simulink model "PositionControlFuzzy"  (R2022b)
settings: Solver=ode3  StartTime=0.0  StopTime=100.0  FixedStep=Ts  RelTol=1e-3
values from neighbouring files (symbols this model uses):
  th_0 = 0    [parte32.m]
  Ts = 100e-3    (= 0.1)    [comparativa.m]    (also in parte32.m)
  x_0 = 0    [parte32.m]
  y_0 = 0    [parte32.m]
undefined symbols (not defined in the file or in its folder): DiscIntNeverNeededParam, sigbuilder_block
libraries: fuzblock x1
settings Model: PacingRate=10  Creator=Edu  LastModifiedBy=rufo
settings SolverCC: AlgebraicLoopSolver=TrustRegion
settings DataIOCC: ReturnWorkspaceOutputs=off
settings DebuggingCC: UnconnectedInputMsg=warning  UnconnectedOutputMsg=warning  UnconnectedLineMsg=warning  SFMachineParentedDataDiag=warning  ArithmeticOperatorsInVariantConditions=warning
settings ModelReferenceCC: EnableRefExpFcnMdlSchedulingChecks=on
settings SFSimCC: CustomCodeUndefinedFunction=UseInterfaceOnly

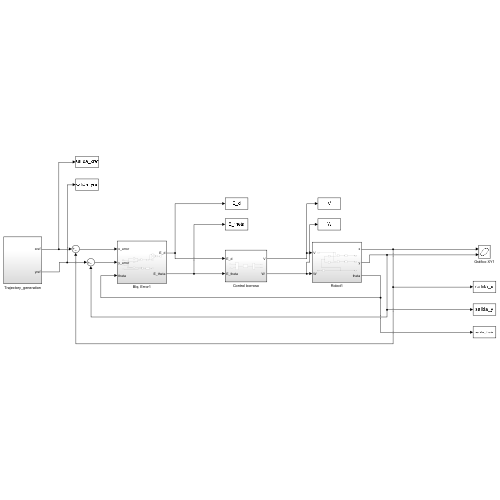
[thumbnail: Simulink's stored preview of the top-level diagram]
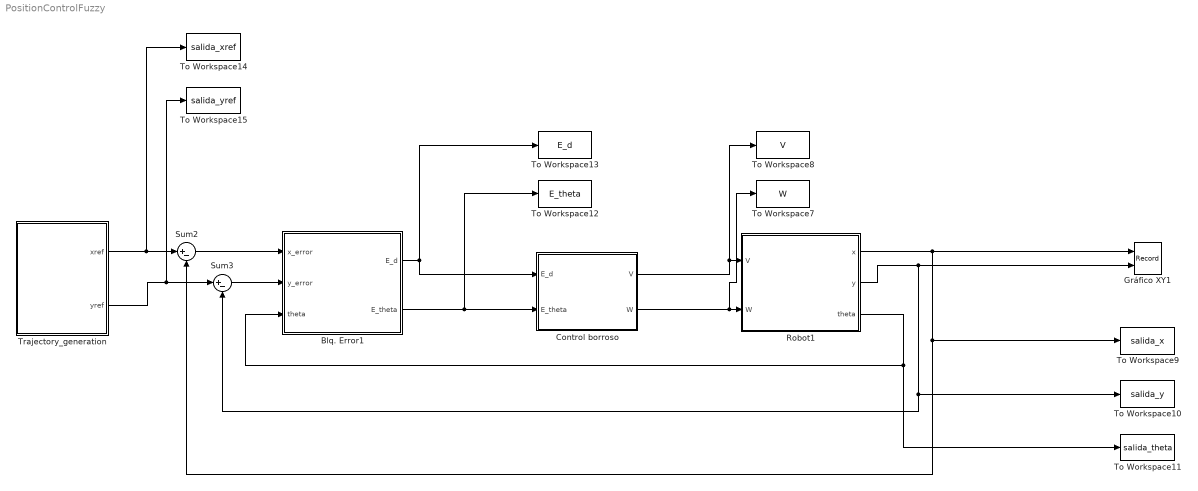
== system PositionControlFuzzy ==
  Blq. Error1 : Subsystem
  Control borroso : Subsystem
  Gráfico XY1 : Record  FileSettingsInternal="{\"entries\":[{\"content\":{\"excelSettings\":{\"content\":{},\"type\":\"Streamout.ExcelSettings\"}},\"type\":\"Streamout.FileSettingStorage\",\"uuid\":\"148716e7-62da-4a17-92fb-a85c316f925a\"}],\"packageUris\":[\"http://schema.mathworks.com/mf0/streamout_blocks/R2020a\"],\"version\":\"1.0\"}"  Layout=[1 1]  SignalsInternal="{\"entries\":[{\"content\":{\"signals\":[{\"content\":{\"blockPath\":[\"PositionControlFuzzy/Gráfico XY1\"],\"channel\":[],\"dimensions\":[1],\"domain\":\"PositionControlFuzzy/Grￃﾡfico XY1\",\"lineColor\":\"#a2142f\",\"plots\":[1],\"port\":1,\"sid\":[\"\"],\"signalID\":1359,\"signalName\":\"Robot1:1\"},\"type\":\"RecordBlkView.Signal\",\"uuid\":\"64a1cd59-4d77-4e73-8dd8-b24fff99f81d\"},{\"content\":{\"blockPath\":[\"PositionControlFuzzy/Gráfico XY1\"],\"channel\":[],\"dimensions\":[1],\"domain\":\"PositionControlFuzzy/Grￃﾡfico XY1\",\"lineColor\":\"#139fff\",\"plots\":[1],\"port\":2,\"sid\":[\"\"],\"signalID\":1363,\"signalName\":\"Robot1:2\"},\"type\":\"RecordBlkView.Signal\",\"uuid\":\"bc7211c2-bf92-4b6c-aa6f-eb73f9fcbfea\"}]},\"type\":\"RecordBlkView.InputSignals\",\"uuid\":\"ff4ee394-39ff-4ff1-a002-becb146826f1\"}],\"packageUris\":[\"http://schema.mathworks.com/mf0/streamout_blocks/R2020a\"],\"version\":\"1.0\"}"  VisualizationBindings="{\"xyplotplugin\":{\"info\":[{\"series\":[{\"bindingParametersList\":[{\"parameter\":\"X-Axis\",\"signalID\":1359,\"signalName\":\"Robot1:1\"},{\"parameter\":\"Y-Axis\",\"signalID\":1363,\"signalName\":\"Robot1:2\"}],\"seriesID\":12570}],\"subplotID\":1}]}}"  CompatibilityTag=XY  st=-1
  Robot1 : Subsystem
  Sum2 : Sum  Inputs=|+-
  Sum3 : Sum  Inputs=|+-
  To Workspace10 : ToWorkspace  VariableName=salida_y  SaveFormat=Structure With Time  SampleTime=-1
  To Workspace11 : ToWorkspace  VariableName=salida_theta  SaveFormat=Structure With Time  SampleTime=-1
  To Workspace12 : ToWorkspace  VariableName=E_theta  SaveFormat=Structure With Time  SampleTime=-1
  To Workspace13 : ToWorkspace  VariableName=E_d  SaveFormat=Structure With Time  SampleTime=-1
  To Workspace14 : ToWorkspace  VariableName=salida_xref  SaveFormat=Structure With Time  SampleTime=-1
  To Workspace15 : ToWorkspace  VariableName=salida_yref  SaveFormat=Structure With Time  SampleTime=-1
  To Workspace7 : ToWorkspace  VariableName=W  SaveFormat=Structure With Time  SampleTime=-1
  To Workspace8 : ToWorkspace  VariableName=V  SaveFormat=Structure With Time  SampleTime=-1
  To Workspace9 : ToWorkspace  VariableName=salida_x  SaveFormat=Structure With Time  SampleTime=-1
  Trajectory_generation : Subsystem
  wires:
  Trajectory_generation/2(yref) -> To Workspace15/1, Sum3/1
  Blq. Error1/1(E_d) -> Control borroso/1("E_d "), To Workspace13/1
  Trajectory_generation/1(xref) -> To Workspace14/1, Sum2/1
  Robot1/2(y) -> Gráfico XY1/2, To Workspace10/1, Sum3/2
  Sum2/1 -> Blq. Error1/1(x_error)
  Blq. Error1/2(E_theta) -> Control borroso/2(E_theta), To Workspace12/1
  Robot1/3(theta) -> Blq. Error1/3(theta), To Workspace11/1
  Robot1/1(x) -> Gráfico XY1/1, To Workspace9/1, Sum2/2
  Sum3/1 -> Blq. Error1/2(y_error)
  Control borroso/1(V) -> To Workspace8/1, Robot1/1(V)
  Control borroso/2("W ") -> To Workspace7/1, Robot1/2(W)

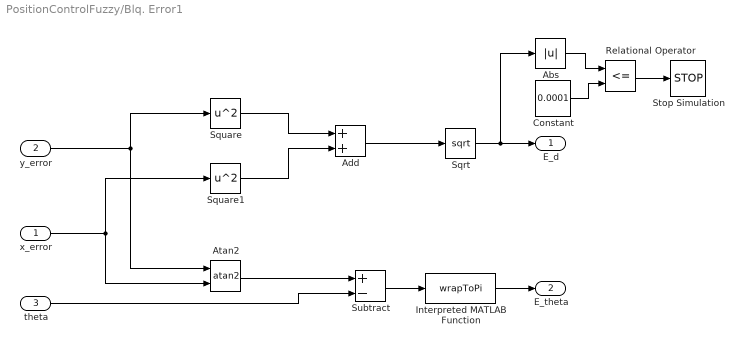
== system PositionControlFuzzy/Blq. Error1 ==
  x_error : Inport
  y_error : Inport  Port=2
  theta : Inport  Port=3
  Abs : Abs  SaturateOnIntegerOverflow=off
  Add : Sum
  Atan2 : Trigonometry  Operator=atan2
  Constant : Constant  Value=0.0001
  Interpreted MATLAB Function : MATLABFcn  MATLABFcn=wrapToPi
  Relational Operator : RelationalOperator  Operator=<=  OutDataTypeStr=boolean  RndMeth=Simplest  InputSameDT=off
  Sqrt : Sqrt
  Square : Math  Operator=square  SignedPower=on
  Square1 : Math  Operator=square  SignedPower=on
  Stop Simulation : Stop
  Subtract : Sum  Inputs=+-  OutMin=[-3.14]  OutMax=[3.14]
  E_d : Outport  VectorParamsAs1DForOutWhenUnconnected=off
  E_theta : Outport  Port=2  OutMin=[-pi]  OutMax=[pi]  VectorParamsAs1DForOutWhenUnconnected=off
  wires:
  y_error/1 -> Atan2/1, Square/1
  x_error/1 -> Atan2/2, Square1/1
  Square/1 -> Add/1
  Square1/1 -> Add/2
  Add/1 -> Sqrt/1
  Sqrt/1 -> Abs/1, E_d/1
  Atan2/1 -> Subtract/1
  theta/1 -> Subtract/2
  Abs/1 -> Relational Operator/1
  Constant/1 -> Relational Operator/2
  Relational Operator/1 -> Stop Simulation/1
  Interpreted MATLAB Function/1 -> E_theta/1
  Subtract/1 -> Interpreted MATLAB Function/1

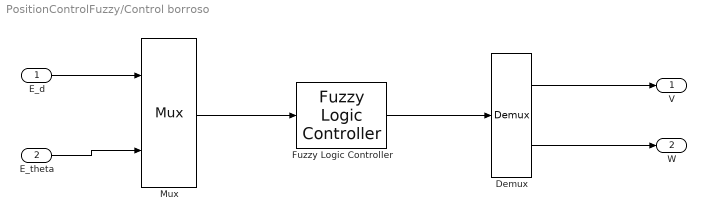
== system PositionControlFuzzy/Control borroso ==
  "E_d " : Inport
  E_theta : Inport  Port=2
  Demux : Demux  Outputs=2
  Fuzzy Logic Controller : fuzblock/Fuzzy Logic  Controller  FIS='borrosoexp.fis'  OutputSampleNumber=101  DataType=double  FuzzifiedInputs=off  RuleFiringStrengths=off  RuleOutputs=off  AggregatedOutputs=off  SimulateUsing=Interpreted execution  OutOfRangeInputValueMessage=warning  NoRuleFiredMessage=warning  EmptyOutputFuzzySetMessage=warning
  Mux : Mux  Inputs=2
  V : Outport  VectorParamsAs1DForOutWhenUnconnected=off
  "W " : Outport  Port=2  VectorParamsAs1DForOutWhenUnconnected=off
  wires:
  Mux/1 -> Fuzzy Logic Controller/1
  "E_d "/1 -> Mux/1
  Demux/1 -> V/1
  Demux/2 -> "W "/1
  E_theta/1 -> Mux/2
  Fuzzy Logic Controller/1 -> Demux/1

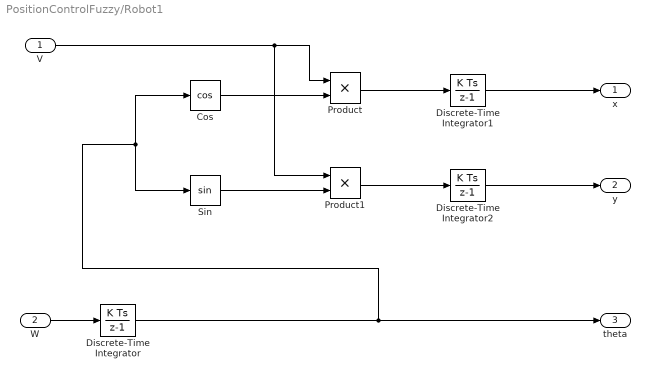
== system PositionControlFuzzy/Robot1 ==
  V : Inport
  W : Inport  Port=2
  Cos : Trigonometry  Operator=cos
  Discrete-Time Integrator : DiscreteIntegrator  SampleTime=-1  ICPrevOutput=DiscIntNeverNeededParam  ICPrevScaledInput=DiscIntNeverNeededParam
  Discrete-Time Integrator1 : DiscreteIntegrator  InitialCondition=-1  SampleTime=-1  ICPrevOutput=DiscIntNeverNeededParam  ICPrevScaledInput=DiscIntNeverNeededParam
  Discrete-Time Integrator2 : DiscreteIntegrator  InitialCondition=-1  SampleTime=-1  ICPrevOutput=DiscIntNeverNeededParam  ICPrevScaledInput=DiscIntNeverNeededParam
  Product : Product
  Product1 : Product
  Sin : Trigonometry
  x : Outport  VectorParamsAs1DForOutWhenUnconnected=off
  y : Outport  Port=2  VectorParamsAs1DForOutWhenUnconnected=off
  theta : Outport  Port=3  VectorParamsAs1DForOutWhenUnconnected=off
  wires:
  Sin/1 -> Product1/2
  Product1/1 -> Discrete-Time Integrator2/1
  Product/1 -> Discrete-Time Integrator1/1
  Discrete-Time Integrator2/1 -> y/1
  V/1 -> Product1/1, Product/1
  Discrete-Time Integrator1/1 -> x/1
  Discrete-Time Integrator/1 -> theta/1, Sin/1, Cos/1
  W/1 -> Discrete-Time Integrator/1
  Cos/1 -> Product/2

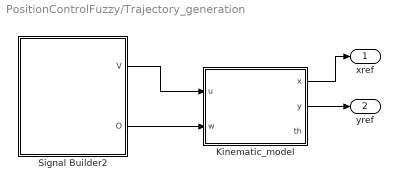
== system PositionControlFuzzy/Trajectory_generation ==
  Kinematic_model : Subsystem
  Signal Builder2 : Subsystem  Tag=STV Subsys  LoadFcn=sigbuilder_block('load');  StartFcn=sigbuilder_block('start');  StopFcn=sigbuilder_block('stop');  ClipboardFcn=sigbuilder_block('clipboard');  mask(Sigbuilder block){tuvar=[0:10]}
      mask help: Sigbuilder GUI
      mask init:
      | if ~strcmp(get_param(bdroot(gcbh),'SimulationStatus'),'stopped') tuvar = sigbuilder_block('maskInit'); end
      settings: CopyFcn=sigbuilder_block('copy');  DeleteFcn=sigbuilder_block('delete');  ModelCloseFcn=sigbuilder_block('modelClose');  PreSaveFcn=sigbuilder_block('preSave');  PauseFcn=sigbuilder_block('pause')  ContinueFcn=sigbuilder_block('continue')  NameChangeFcn=sigbuilder_block('namechange');  OpenFcn=sigbuilder_block('open',[60 45 534.4 467.25 ]);  CloseFcn=sigbuilder_block('close');
      mask Display: plot(0, 0, 100, 100,[2, 2, 32, 32, 2], [68, 8, 8, 68, 68],[32, 2], [38, 38], [32, 19, 2],[53, 60, 44], [32, 17, 17, 2],[16, 16, 31, 31]);txt = getActiveGroup(gcbh);text(2, 100, txt,'verticalAlignment', 'top');
  xref : Outport  VectorParamsAs1DForOutWhenUnconnected=off
  yref : Outport  Port=2  VectorParamsAs1DForOutWhenUnconnected=off
  wires:
  Kinematic_model/2(y) -> yref/1
  Kinematic_model/1(x) -> xref/1
  Signal Builder2/2(O) -> Kinematic_model/2(w)
  Signal Builder2/1(V) -> Kinematic_model/1(u)

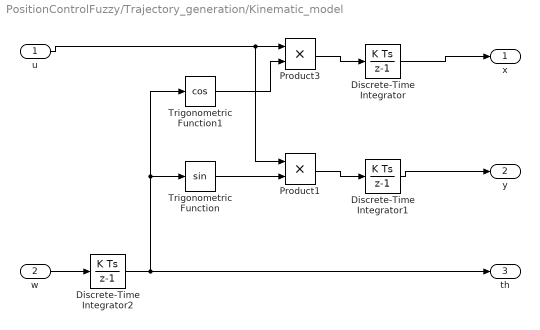
== system PositionControlFuzzy/Trajectory_generation/Kinematic_model ==
  u : Inport
  w : Inport  Port=2
  Discrete-Time Integrator : DiscreteIntegrator  InitialCondition=x_0  SampleTime=Ts  ICPrevOutput=DiscIntNeverNeededParam  ICPrevScaledInput=DiscIntNeverNeededParam
  Discrete-Time Integrator1 : DiscreteIntegrator  InitialCondition=y_0  SampleTime=Ts  ICPrevOutput=DiscIntNeverNeededParam  ICPrevScaledInput=DiscIntNeverNeededParam
  Discrete-Time Integrator2 : DiscreteIntegrator  InitialCondition=th_0  SampleTime=Ts  ICPrevOutput=DiscIntNeverNeededParam  ICPrevScaledInput=DiscIntNeverNeededParam
  Product1 : Product
  Product3 : Product
  Trigonometric Function : Trigonometry
  Trigonometric Function1 : Trigonometry  Operator=cos
  x : Outport  VectorParamsAs1DForOutWhenUnconnected=off
  y : Outport  Port=2  VectorParamsAs1DForOutWhenUnconnected=off
  th : Outport  Port=3  VectorParamsAs1DForOutWhenUnconnected=off
  wires:
  Discrete-Time Integrator/1 -> x/1
  Discrete-Time Integrator1/1 -> y/1
  Trigonometric Function1/1 -> Product3/2
  u/1 -> Product3/1, Product1/1
  Trigonometric Function/1 -> Product1/2
  w/1 -> Discrete-Time Integrator2/1
  Product3/1 -> Discrete-Time Integrator/1
  Product1/1 -> Discrete-Time Integrator1/1
  Discrete-Time Integrator2/1 -> th/1, Trigonometric Function/1, Trigonometric Function1/1

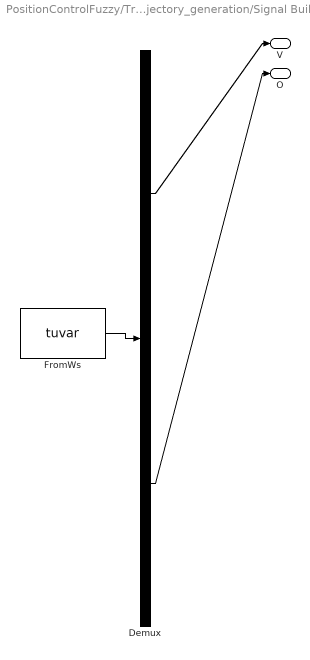
== system PositionControlFuzzy/Trajectory_generation/Signal Builder2 ==
  Demux : Demux  Tag=STV Demux  Outputs=2
      settings: DisplayOption=none
  FromWs : FromWorkspace  Tag=STV FromWs  VariableName=tuvar
      SigBuilderData=|
      | common.afterFinalStr = 'Extrapolate'
      | common.sampleTime = '0'
      | dataSet.timeRange = [0 115]
      | dataSet.name = 'Group 1'
      | sbobj.Groups.Name = 'Group 1'
      | sbobj.Groups.Signals(1).Name = 'V'
      | sbobj.Groups.Signals(1).XData = [0 87 87 115]
      | sbobj.Groups.Signals(1).YData = [0.25 0.25 0 0]
      | sbobj.Groups.Signals(2).Name = 'O'
      | sbobj.Groups.Signals(2).XData = [0 12 12 30.849 30.849 55.981 55.981 74.83 74.83 99.962 115]
      | sbobj.Groups.Signals(2).YData = [0 0 0.25 0.25 -0.25 -0.25 0.25 0.25 0 0 0]
      | sbobj.Groups.TimeRange = [0 115]
  V : Outport  Tag=STV Outport  VectorParamsAs1DForOutWhenUnconnected=off
  O : Outport  Tag=STV Outport  Port=2  VectorParamsAs1DForOutWhenUnconnected=off
  wires:
  Demux/2 -> O/1
  Demux/1 -> V/1
  FromWs/1 -> Demux/1
